simulink model "simQuad"  (R2016a)
settings: Solver=VariableStepAuto  StartTime=0.0  StopTime=10  FixedStep=dt  RelTol=1e-3
values from neighbouring files (symbols this model uses):
  ic = [-3 0 0 0 0 0 0 0 0 0 0 0]    [cf_pid_compare.m]    (also in main.m = [0 0 0 0 0 0 0 0 0 0 0 0])
  Ki = 0.004    [main.m]
  Kp = 0.5    [main.m]
  r2d = 180/pi    (= 57.2957795131)    [main.m]
  T_takeoff = 5    [main.m]
undefined symbols (not defined in the file or in its folder): default_ctl, run_away
undefined symbols (not defined in the file): cf2, geometric_ctl, ic2
libraries: simulink x22, aerolibtransform2 x10, vrlib x8, aerolibutil x5, cstblocks x4, aerolibnav x2, dspmathops x2
(part 1 of 2)
settings Model: Creator=appatte2  LastModifiedBy=arun

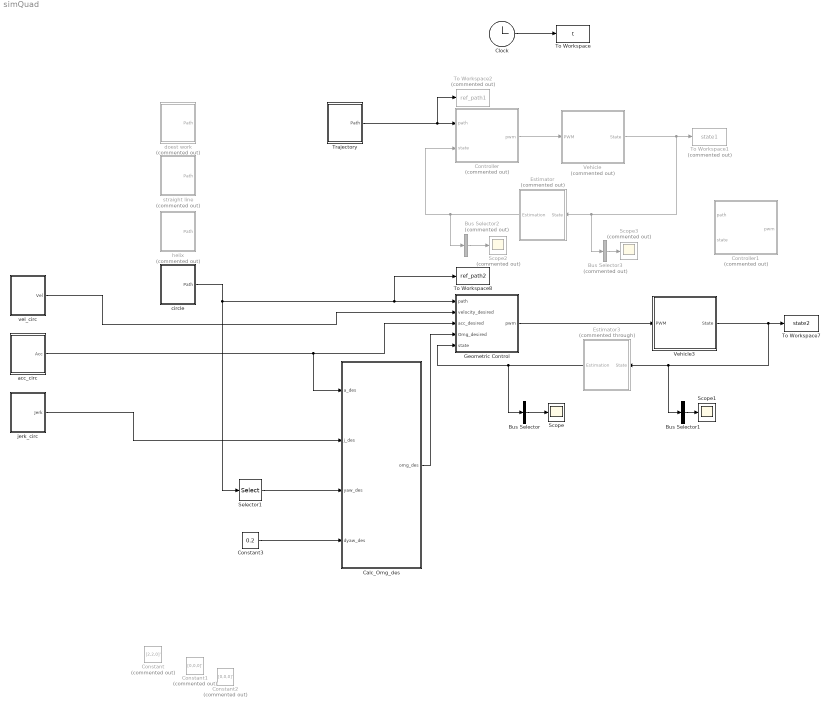
== system simQuad ==
  Bus Selector : BusSelector  OutputSignals=roll,pitch,yaw  OutputAsBus=on
  Bus Selector1 : BusSelector  OutputSignals=roll,pitch,yaw  OutputAsBus=on
  Bus Selector2 : BusSelector  Commented=on  OutputSignals=roll,pitch,yaw  OutputAsBus=on
  Bus Selector3 : BusSelector  Commented=on  OutputSignals=roll,pitch,yaw  OutputAsBus=on
  "Calc_Omg_des " : MATLAB Function  TreatAsAtomicUnit=on
  Clock : Clock
  Constant : Constant  Commented=on  Value=[2,2,0]'
  Constant1 : Constant  Commented=on  Value=[0,0,0]'
  Constant2 : Constant  Commented=on  Value=[0,0,0]'
  Constant3 : Constant  Value=0.2
  Controller : Subsystem  Commented=on  mask(PID Controller for Quadrotor){mix=default_ctl.mix, rates=default_ctl.rates, att=default_ctl.att, pos=default_ctl.pos, sat=default_ctl.sat, intSat=default_ctl.intSat}
      mask prompts: mix "Motor Mixing Table"; rates "Rate Control Table"; att "Attitude Control Table"; pos "Position Control Table"; sat "Attitude Limits"; intSat "Integral Saturation"
      mask help: Allows user to set parameters for pid controllers on rates, angles and linear position.
  Controller1 : Subsystem  Commented=on  mask(PID Controller for Quadrotor){mix=default_ctl.mix, rates=default_ctl.rates, att=default_ctl.att, pos=default_ctl.pos, sat=default_ctl.sat, intSat=default_ctl.intSat}
      mask prompts: mix "Motor Mixing Table"; rates "Rate Control Table"; att "Attitude Control Table"; pos "Position Control Table"; sat "Attitude Limits"; intSat "Integral Saturation"
      mask help: Allows user to set parameters for pid controllers on rates, angles and linear position.
  Estimator : Subsystem  Commented=on  mask{rng_seed=1111}
      mask prompts: rng_seed "Random Seed"
  Estimator3 : Subsystem  Commented=through  mask{rng_seed=1111}
      mask prompts: rng_seed "Random Seed"
  Geometric Control : Subsystem  mask(PID Controller for Quadrotor){model=cf2, ctl=geometric_ctl}
      mask prompts: model "Quad Model"; ctl "Controller"
      mask help: Allows user to set parameters for pid controllers on rates, angles and linear position.
  Scope : Scope
  Scope1 : Scope
  Scope2 : Scope  Commented=on
  Scope3 : Scope  Commented=on
  Selector1 : Selector  InputPortWidth=4  IndexOptions=Index vector (dialog)  Indices=[4]  OutputSizes=1
  To Workspace : ToWorkspace  VariableName=t  SaveFormat=Timeseries  SampleTime=-1
  To Workspace1 : ToWorkspace  Commented=on  VariableName=state1  SampleTime=-1
  To Workspace2 : ToWorkspace  Commented=on  VariableName=ref_path1  SampleTime=-1
      settings: Save2DSignal=2-D array (concatenate along first dimension)
  To Workspace7 : ToWorkspace  VariableName=state2  SampleTime=-1
  To Workspace8 : ToWorkspace  VariableName=ref_path2  SampleTime=-1
      settings: Save2DSignal=2-D array (concatenate along first dimension)
  Trajectory : Subsystem
  Vehicle : Subsystem  Commented=on  mask{model=cf2, ic=ic}
      mask prompts: model "Model Object"; ic "Initial Condition"
  Vehicle3 : Subsystem  mask{model=cf2, ic=ic2}
      mask prompts: model "Model Object"; ic "Initial Condition"
  acc_circ : Subsystem
  "circle " : Subsystem
  doest work : Subsystem  Commented=on
  helix : Subsystem  Commented=on
  jerk_circ : Subsystem
  straight line : Subsystem  Commented=on
  vel_circ : Subsystem
  wires:
  Clock/1 -> To Workspace/1
  Controller/1(pwm) -> Vehicle/1(PWM)
  Geometric Control/1(pwm) -> Vehicle3/1(PWM)
  Trajectory/1(Path) -> To Workspace2/1, Controller/1(path)
  "Calc_Omg_des "/1(omg_des) -> Geometric Control/4(Omg_desired)
  Estimator3/1(Estimation) -> Geometric Control/5(state), Bus Selector/1
  Vehicle3/1(State) -> Estimator3/1(State), Bus Selector1/1, To Workspace7/1
  Bus Selector/1 -> Scope/1
  Bus Selector1/1 -> Scope1/1
  Estimator/1(Estimation) -> Bus Selector2/1, Controller/2(state)
  Bus Selector2/1 -> Scope2/1
  Vehicle/1(State) -> Bus Selector3/1, Estimator/1(State), To Workspace1/1
  Bus Selector3/1 -> Scope3/1
  "circle "/1(Path) -> To Workspace8/1, Geometric Control/1(path), Selector1/1
  Selector1/1 -> "Calc_Omg_des "/3(yaw_des)
  Constant3/1 -> "Calc_Omg_des "/4(dyaw_des)
  vel_circ/1(Vel) -> Geometric Control/2(velocity_desired)
  acc_circ/1(Acc) -> "Calc_Omg_des "/1(a_des), Geometric Control/3("acc_desired ")
  jerk_circ/1(Jerk) -> "Calc_Omg_des "/2(j_des)

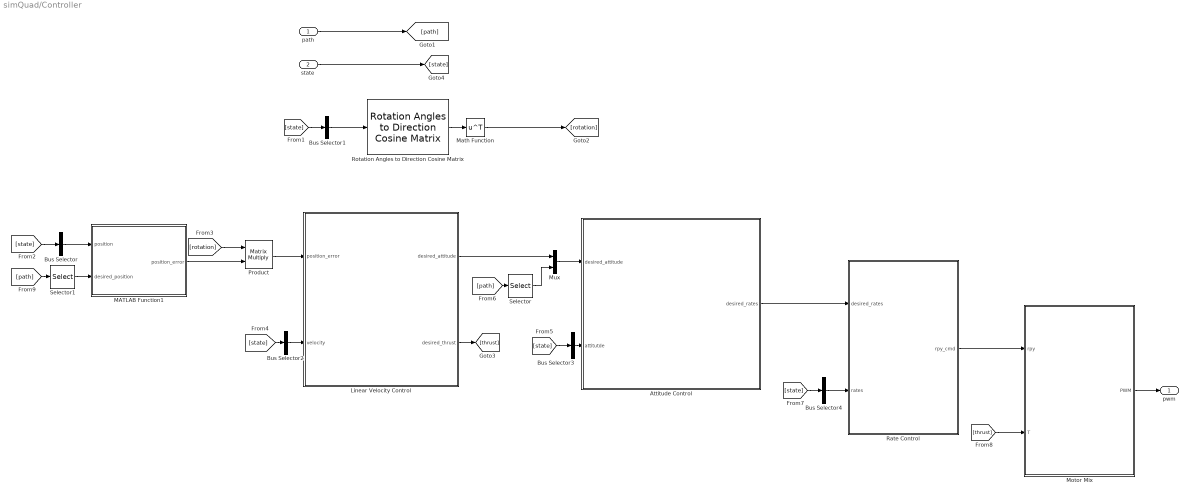
== system simQuad/Controller ==
  path : Inport
  state : Inport  Port=2
  Attitude Control : Subsystem
  Bus Selector : BusSelector  OutputSignals=x,y,z  OutputAsBus=on
  Bus Selector1 : BusSelector  OutputSignals=roll,pitch,yaw  OutputAsBus=on
  Bus Selector2 : BusSelector  OutputSignals=dx,dy,dz  OutputAsBus=on
  Bus Selector3 : BusSelector  OutputSignals=roll,pitch,yaw  OutputAsBus=on
  Bus Selector4 : BusSelector  OutputSignals=droll,dpitch,dyaw  OutputAsBus=on
  Linear Velocity Control : Subsystem
  MATLAB Function1 : MATLAB Function  TreatAsAtomicUnit=on
  Math Function : Math  Operator=transpose  SaturateOnIntegerOverflow=on
  Motor Mix : Subsystem
  Mux : Mux  Inputs=2
  Product : Product  Multiplication=Matrix(*)
  Rate Control : Subsystem
  Rotation Angles to Direction Cosine Matrix : aerolibtransform2/Rotation Angles to Direction Cosine Matrix  rotationOrder=ZYX
  Selector : Selector  InputPortWidth=4  IndexOptions=Index vector (dialog)  Indices=[4]  OutputSizes=1
  Selector1 : Selector  InputPortWidth=4  IndexOptions=Index vector (dialog)  Indices=[1 2 3]  OutputSizes=1
  pwm : Outport
  wires:
  [path] -> Selector1/1
  [state] -> Bus Selector/1
  Motor Mix/1(PWM) -> pwm/1
  Selector1/1 -> MATLAB Function1/2(desired_position)
  Bus Selector/1 -> MATLAB Function1/1(position)
  [rotation] -> Product/1
  Mux/1 -> Attitude Control/1(desired_attitude)
  Bus Selector1/1 -> Rotation Angles to Direction Cosine Matrix/1
  [state] -> Bus Selector3/1
  Bus Selector3/1 -> Attitude Control/2(attitutde)
  Bus Selector2/1 -> Linear Velocity Control/2(velocity)
  [state] -> Bus Selector2/1
  [state] -> Bus Selector1/1
  [thrust] -> Motor Mix/2(T)
  Attitude Control/1(desired_rates) -> Rate Control/1(desired_rates)
  [state] -> Bus Selector4/1
  Bus Selector4/1 -> Rate Control/2(rates)
  [path] -> Selector/1
  Selector/1 -> Mux/2
  Linear Velocity Control/2(desired_thrust) -> [thrust]
  state/1 -> [state]
  path/1 -> [path]
  MATLAB Function1/1(position_error) -> Product/2
  Rotation Angles to Direction Cosine Matrix/1 -> Math Function/1
  Product/1 -> Linear Velocity Control/1(position_error)
  Linear Velocity Control/1(desired_attitude) -> Mux/1
  Math Function/1 -> [rotation]
  Rate Control/1(rpy_cmd) -> Motor Mix/1(rpy)

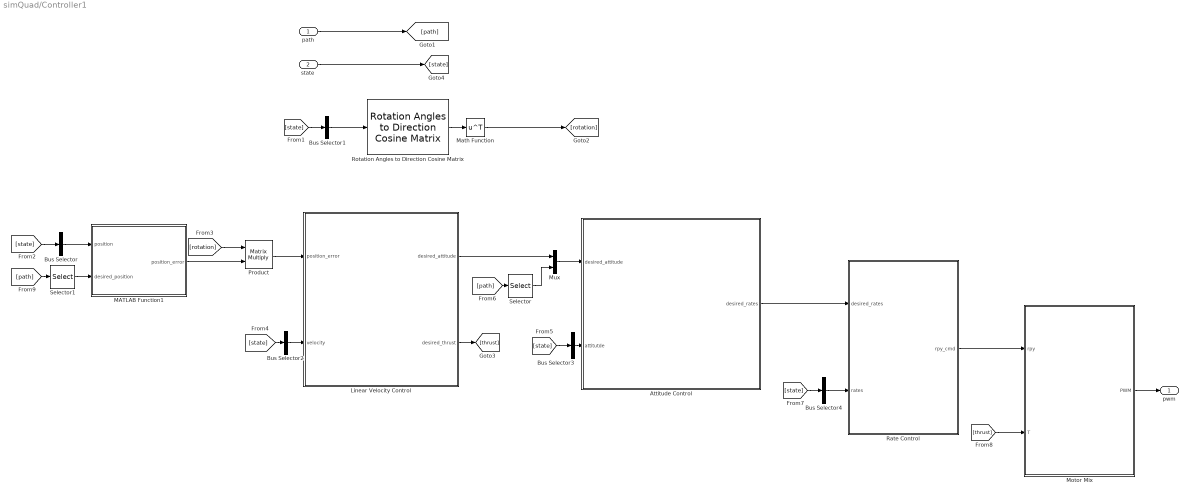
== system simQuad/Controller1 ==
  path : Inport
  state : Inport  Port=2
  Attitude Control : Subsystem
  Bus Selector : BusSelector  OutputSignals=x,y,z  OutputAsBus=on
  Bus Selector1 : BusSelector  OutputSignals=roll,pitch,yaw  OutputAsBus=on
  Bus Selector2 : BusSelector  OutputSignals=dx,dy,dz  OutputAsBus=on
  Bus Selector3 : BusSelector  OutputSignals=roll,pitch,yaw  OutputAsBus=on
  Bus Selector4 : BusSelector  OutputSignals=droll,dpitch,dyaw  OutputAsBus=on
  Linear Velocity Control : Subsystem
  MATLAB Function1 : MATLAB Function  TreatAsAtomicUnit=on
  Math Function : Math  Operator=transpose  SaturateOnIntegerOverflow=on
  Motor Mix : Subsystem
  Mux : Mux  Inputs=2
  Product : Product  Multiplication=Matrix(*)
  Rate Control : Subsystem
  Rotation Angles to Direction Cosine Matrix : aerolibtransform2/Rotation Angles to Direction Cosine Matrix  rotationOrder=ZYX
  Selector : Selector  InputPortWidth=4  IndexOptions=Index vector (dialog)  Indices=[4]  OutputSizes=1
  Selector1 : Selector  InputPortWidth=4  IndexOptions=Index vector (dialog)  Indices=[1 2 3]  OutputSizes=1
  pwm : Outport
  wires:
  [path] -> Selector1/1
  [state] -> Bus Selector/1
  Motor Mix/1(PWM) -> pwm/1
  Selector1/1 -> MATLAB Function1/2(desired_position)
  Bus Selector/1 -> MATLAB Function1/1(position)
  [rotation] -> Product/1
  Mux/1 -> Attitude Control/1(desired_attitude)
  Bus Selector1/1 -> Rotation Angles to Direction Cosine Matrix/1
  [state] -> Bus Selector3/1
  Bus Selector3/1 -> Attitude Control/2(attitutde)
  Bus Selector2/1 -> Linear Velocity Control/2(velocity)
  [state] -> Bus Selector2/1
  [state] -> Bus Selector1/1
  [thrust] -> Motor Mix/2(T)
  Attitude Control/1(desired_rates) -> Rate Control/1(desired_rates)
  [state] -> Bus Selector4/1
  Bus Selector4/1 -> Rate Control/2(rates)
  [path] -> Selector/1
  Selector/1 -> Mux/2
  Linear Velocity Control/2(desired_thrust) -> [thrust]
  state/1 -> [state]
  path/1 -> [path]
  MATLAB Function1/1(position_error) -> Product/2
  Rotation Angles to Direction Cosine Matrix/1 -> Math Function/1
  Product/1 -> Linear Velocity Control/1(position_error)
  Linear Velocity Control/1(desired_attitude) -> Mux/1
  Math Function/1 -> [rotation]
  Rate Control/1(rpy_cmd) -> Motor Mix/1(rpy)

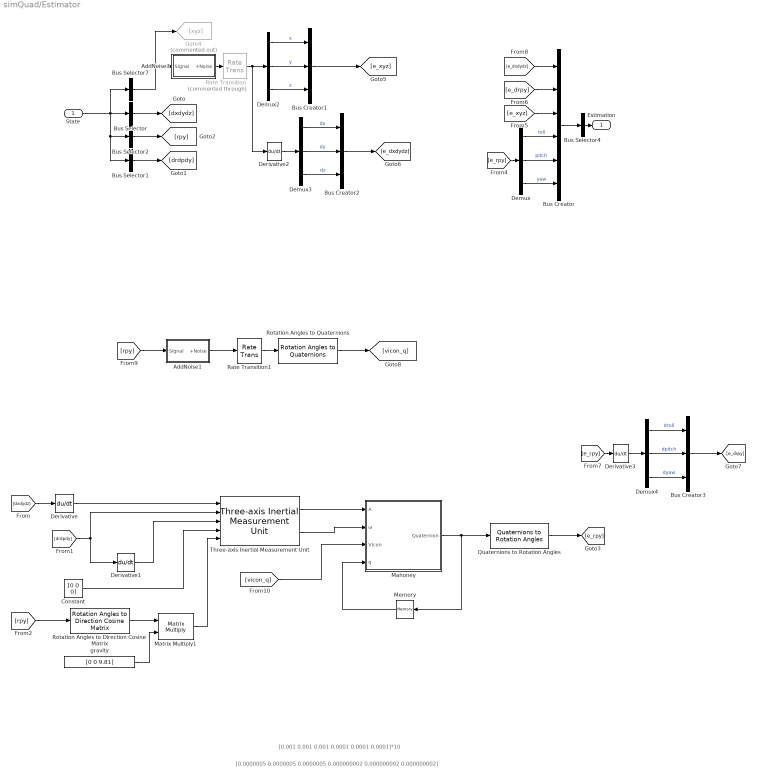
== system simQuad/Estimator ==
  note: [0.001 0.001 0.001 0.0001 0.0001 0.0001]*10
  note: [0.0000005 0.0000005 0.0000005 0.000000002 0.000000002 0.000000002]
  State : Inport
  AddNoise1 : Subsystem
  AddNoise3 : Subsystem
  Bus Creator : BusCreator  Inputs=6
  Bus Creator1 : BusCreator  Inputs=3
  Bus Creator2 : BusCreator  Inputs=3
  Bus Creator3 : BusCreator  Inputs=3
  Bus Selector : BusSelector  OutputSignals=dx,dy,dz  OutputAsBus=on
  Bus Selector1 : BusSelector  OutputSignals=droll,dpitch,dyaw  OutputAsBus=on
  Bus Selector2 : BusSelector  OutputSignals=roll,pitch,yaw  OutputAsBus=on
  Bus Selector4 : BusSelector  OutputSignals=roll,pitch,yaw,signal3.x,signal3.y,signal3.z,signal2.droll,signal2.dpitch,signal2.dyaw,signal1.dx,signal1.dy,signal1.dz  OutputAsBus=on
  Bus Selector7 : BusSelector  OutputSignals=x,y,z  OutputAsBus=on
  Constant : Constant  Value=[0 0 0]
  Demux{,2..4} (4 alike) : Demux  Outputs=3
  Derivative{,1..3} (4 alike) : Derivative
  Goto4 : Goto  Commented=on  GotoTag=xyz
  Mahoney : Subsystem
  Matrix Multiply1 : Product  Multiplication=Matrix(*)
  Memory : Memory  X0=[1 0 0 0]
  Quaternions to Rotation Angles : aerolibtransform2/Quaternions to Rotation Angles  rotationOrder=XYZ
  Rate Transition : RateTransition  Commented=through  OutPortSampleTime=0.005
  Rate Transition1 : RateTransition  OutPortSampleTime=0.005
  Rotation Angles to Direction Cosine Matrix : aerolibtransform2/Rotation Angles to Direction Cosine Matrix  rotationOrder=XYZ
  Rotation Angles to Quaternions : aerolibtransform2/Rotation Angles to Quaternions  rotationOrder=XYZ
  Three-axis Inertial Measurement Unit : aerolibnav/Three-axis Inertial Measurement Unit  units=Metric (MKS)  imu=[0 0 0]  dtype_a=on  w_a=190  z_a=0.707  a_sf_cc=[0.98 0 0; 0 0.98 0; 0 0 0.98]  a_bias=[0 0 0]  a_sat="[-19.62  -19.62  -19.62 19.62 19.62 19.62]"  dtype_g=on  w_g=190  z_g=0.707  g_sf_cc=[.98 0 0; 0 .98 0; 0 0 .98]  g_bias=[0 0 0]  g_sens=[0 0 0]  g_sat="[-4.36  -4.36  -4.36 4.36 4.36 4.36]"  i_rand=on  i_seeds=[23093 23094 23095 23096 23097 23098]*rng_seed  i_pow=[0.001 0.001 0.001 0.0001 0.0001 0.0001]*10  i_Ts=0
  gravity : Constant  Value=[0 0 9.81]
  Estimation : Outport
  wires:
  State/1 -> Bus Selector1/1, Bus Selector2/1, Bus Selector7/1, Bus Selector/1
  Bus Creator/1 -> Bus Selector4/1
  Derivative/1 -> Three-axis Inertial Measurement Unit/1
  Constant/1 -> Three-axis Inertial Measurement Unit/4
  Memory/1 -> Mahoney/4(q)
  Mahoney/1(Quaternion) -> Memory/1, Quaternions to Rotation Angles/1
  Three-axis Inertial Measurement Unit/1 -> Mahoney/1(A)
  Three-axis Inertial Measurement Unit/2 -> Mahoney/2(ω)
  Derivative1/1 -> Three-axis Inertial Measurement Unit/3
  gravity/1 -> Matrix Multiply1/2
  Rotation Angles to Direction Cosine Matrix/1 -> Matrix Multiply1/1
  Matrix Multiply1/1 -> Three-axis Inertial Measurement Unit/5
  Bus Selector/1 -> [dxdydz]
  [dxdydz] -> Derivative/1
  Bus Selector1/1 -> [drdpdy]
  [drdpdy] -> Three-axis Inertial Measurement Unit/2, Derivative1/1
  Bus Selector2/1 -> [rpy]
  [rpy] -> Rotation Angles to Direction Cosine Matrix/1
  Demux/2 -> Bus Creator/5  "pitch"
  Demux/1 -> Bus Creator/4  "roll"
  [e_rpy] -> Demux/1
  Demux/3 -> Bus Creator/6  "yaw"
  Bus Selector4/1 -> Estimation/1
  [e_xyz] -> Bus Creator/3
  [e_drpy] -> Bus Creator/2
  [e_dxdydz] -> Bus Creator/1
  Bus Selector7/1 -> Goto4/1, AddNoise3/1(Signal)
  AddNoise3/1(+Noise) -> Rate Transition/1
  Rate Transition/1 -> Derivative2/1, Demux2/1
  Demux2/1 -> Bus Creator1/1  "x"
  Demux2/3 -> Bus Creator1/3  "z"
  Demux2/2 -> Bus Creator1/2  "y"
  Bus Creator1/1 -> [e_xyz]
  Demux3/3 -> Bus Creator2/3  "dz"
  Derivative2/1 -> Demux3/1
  Demux3/2 -> Bus Creator2/2  "dy"
  Demux3/1 -> Bus Creator2/1  "dx"
  Bus Creator2/1 -> [e_dxdydz]
  Demux4/3 -> Bus Creator3/3  "dyaw"
  Derivative3/1 -> Demux4/1
  Demux4/2 -> Bus Creator3/2  "dpitch"
  Demux4/1 -> Bus Creator3/1  "droll"
  Bus Creator3/1 -> [e_drpy]
  [e_rpy] -> Derivative3/1
  Rotation Angles to Quaternions/1 -> [vicon_q]
  [vicon_q] -> Mahoney/3(Vicon)
  Rate Transition1/1 -> Rotation Angles to Quaternions/1
  AddNoise1/1(+Noise) -> Rate Transition1/1
  [rpy] -> AddNoise1/1(Signal)
  Quaternions to Rotation Angles/1 -> [e_rpy]

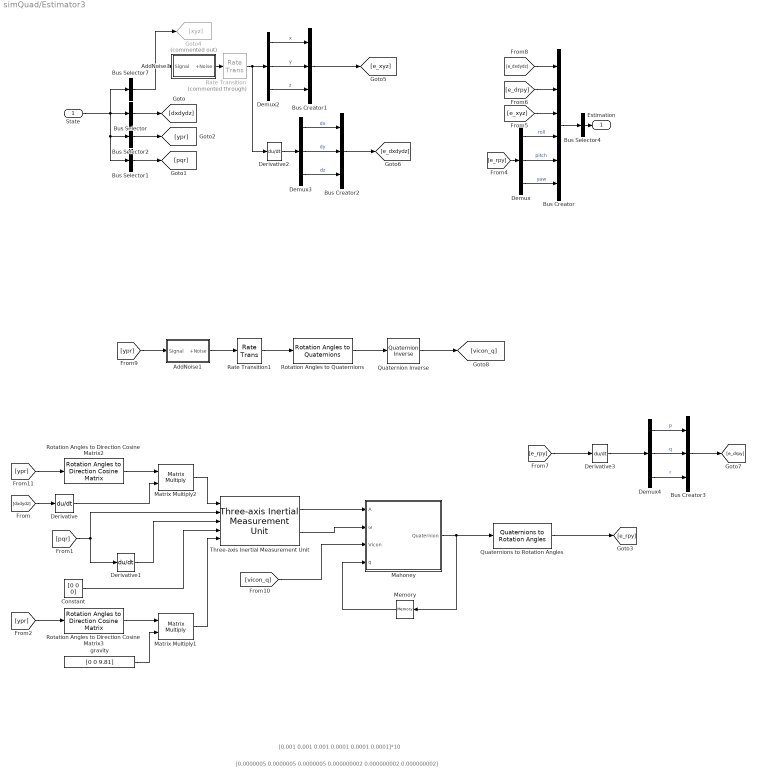
== system simQuad/Estimator3 ==
  note: [0.0000005 0.0000005 0.0000005 0.000000002 0.000000002 0.000000002]
  note: [0.001 0.001 0.001 0.0001 0.0001 0.0001]*10
  State : Inport
  AddNoise1 : Subsystem
  AddNoise3 : Subsystem
  Bus Creator : BusCreator  Inputs=6
  Bus Creator1 : BusCreator  Inputs=3
  Bus Creator2 : BusCreator  Inputs=3
  Bus Creator3 : BusCreator  Inputs=3
  Bus Selector : BusSelector  OutputSignals=dx,dy,dz  OutputAsBus=on
  Bus Selector1 : BusSelector  OutputSignals=p,q,r  OutputAsBus=on
  Bus Selector2 : BusSelector  OutputSignals=yaw,pitch,roll  OutputAsBus=on
  Bus Selector4 : BusSelector  OutputSignals=roll,pitch,yaw,signal3.x,signal3.y,signal3.z,signal2.p,signal2.q,signal2.r,signal1.dx,signal1.dy,signal1.dz  OutputAsBus=on
  Bus Selector7 : BusSelector  OutputSignals=x,y,z  OutputAsBus=on
  Constant : Constant  Value=[0 0 0]
  Demux{,2..4} (4 alike) : Demux  Outputs=3
  Derivative{,1..3} (4 alike) : Derivative
  Goto4 : Goto  Commented=on  GotoTag=xyz
  Mahoney : Subsystem
  Matrix Multiply1 : Product  Multiplication=Matrix(*)
  Matrix Multiply2 : Product  Multiplication=Matrix(*)
  Memory : Memory  X0=[1 0 0 0]
  Quaternion Inverse : aerolibutil/Quaternion Inverse
  Quaternions to Rotation Angles : aerolibtransform2/Quaternions to Rotation Angles  rotationOrder=XYZ
  Rate Transition : RateTransition  Commented=through  OutPortSampleTime=0.005
  Rate Transition1 : RateTransition  OutPortSampleTime=0.005
  Rotation Angles to Direction Cosine Matrix2 : aerolibtransform2/Rotation Angles to Direction Cosine Matrix  rotationOrder=ZYX
  Rotation Angles to Direction Cosine Matrix3 : aerolibtransform2/Rotation Angles to Direction Cosine Matrix  rotationOrder=ZYX
  Rotation Angles to Quaternions : aerolibtransform2/Rotation Angles to Quaternions  rotationOrder=ZYX
  Three-axis Inertial Measurement Unit : aerolibnav/Three-axis Inertial Measurement Unit  units=Metric (MKS)  imu=[0 0 0]  dtype_a=on  w_a=190  z_a=0.707  a_sf_cc=[0.98 0 0; 0 0.98 0; 0 0 0.98]  a_bias=[0 0 0]  a_sat="[-19.62  -19.62  -19.62 19.62 19.62 19.62]"  dtype_g=on  w_g=190  z_g=0.707  g_sf_cc=[.98 0 0; 0 .98 0; 0 0 .98]  g_bias=[0 0 0]  g_sens=[0 0 0]  g_sat="[-4.36  -4.36  -4.36 4.36 4.36 4.36]"  i_rand=on  i_seeds=[23093 23094 23095 23096 23097 23098]*rng_seed  i_pow=[0.001 0.001 0.001 0.0001 0.0001 0.0001]*10  i_Ts=0
  gravity : Constant  Value=[0 0 9.81]
  Estimation : Outport
  wires:
  [ypr] -> AddNoise1/1(Signal)
  AddNoise1/1(+Noise) -> Rate Transition1/1
  Rate Transition1/1 -> Rotation Angles to Quaternions/1
  [vicon_q] -> Mahoney/3(Vicon)
  [e_rpy] -> Derivative3/1
  Bus Creator3/1 -> [e_drpy]
  Demux4/1 -> Bus Creator3/1  "p"
  Demux4/2 -> Bus Creator3/2  "q"
  Derivative3/1 -> Demux4/1
  Demux4/3 -> Bus Creator3/3  "r"
  Bus Creator2/1 -> [e_dxdydz]
  Demux3/1 -> Bus Creator2/1  "dx"
  Demux3/2 -> Bus Creator2/2  "dy"
  Derivative2/1 -> Demux3/1
  Demux3/3 -> Bus Creator2/3  "dz"
  Bus Creator1/1 -> [e_xyz]
  Demux2/2 -> Bus Creator1/2  "y"
  Demux2/3 -> Bus Creator1/3  "z"
  Demux2/1 -> Bus Creator1/1  "x"
  Rate Transition/1 -> Demux2/1, Derivative2/1
  AddNoise3/1(+Noise) -> Rate Transition/1
  Bus Selector7/1 -> AddNoise3/1(Signal), Goto4/1
  [e_dxdydz] -> Bus Creator/1
  [e_drpy] -> Bus Creator/2
  [e_xyz] -> Bus Creator/3
  Bus Selector4/1 -> Estimation/1
  Demux/3 -> Bus Creator/6  "yaw"
  [e_rpy] -> Demux/1
  Demux/1 -> Bus Creator/4  "roll"
  Demux/2 -> Bus Creator/5  "pitch"
  Bus Selector2/1 -> [ypr]
  [pqr] -> Derivative1/1, Three-axis Inertial Measurement Unit/2
  Bus Selector1/1 -> [pqr]
  [dxdydz] -> Derivative/1
  Bus Selector/1 -> [dxdydz]
  Matrix Multiply1/1 -> Three-axis Inertial Measurement Unit/5
  Rotation Angles to Direction Cosine Matrix3/1 -> Matrix Multiply1/1
  gravity/1 -> Matrix Multiply1/2
  Derivative1/1 -> Three-axis Inertial Measurement Unit/3
  Three-axis Inertial Measurement Unit/2 -> Mahoney/2(ω)
  Three-axis Inertial Measurement Unit/1 -> Mahoney/1(A)
  Memory/1 -> Mahoney/4(q)
  Constant/1 -> Three-axis Inertial Measurement Unit/4
  Derivative/1 -> Matrix Multiply2/2
  Bus Creator/1 -> Bus Selector4/1
  State/1 -> Bus Selector/1, Bus Selector7/1, Bus Selector2/1, Bus Selector1/1
  Matrix Multiply2/1 -> Three-axis Inertial Measurement Unit/1
  Rotation Angles to Direction Cosine Matrix2/1 -> Matrix Multiply2/1
  [ypr] -> Rotation Angles to Direction Cosine Matrix2/1
  [ypr] -> Rotation Angles to Direction Cosine Matrix3/1
  Rotation Angles to Quaternions/1 -> Quaternion Inverse/1
  Mahoney/1(Quaternion) -> Quaternions to Rotation Angles/1, Memory/1
  Quaternions to Rotation Angles/1 -> [e_rpy]
  Quaternion Inverse/1 -> [vicon_q]

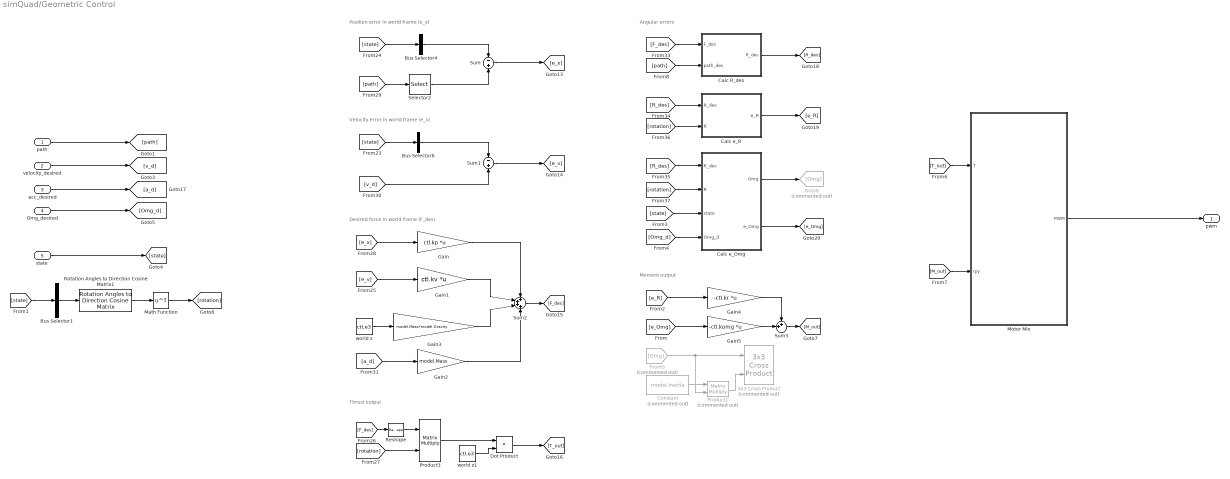
== system simQuad/Geometric Control ==
  note: Moment output
  note: Angular errors
  note: Thrust output
  note: Desired force in world frame (F_des)
  note: Velocity error in world frame (e_v)
  note: Position error in world frame (e_x)
  path : Inport
  velocity_desired : Inport  Port=2
  "acc_desired " : Inport  Port=3
  Omg_desired : Inport  Port=4
  state : Inport  Port=5
  3x3 Cross Product : aerolibutil/3x3 Cross Product  Commented=on
  Bus Selector1 : BusSelector  OutputSignals=yaw,pitch,roll  OutputAsBus=on
  Bus Selector4 : BusSelector  OutputSignals=x,y,z  OutputAsBus=on
  Bus Selector6 : BusSelector  OutputSignals=dx,dy,dz  OutputAsBus=on
  Calc R_des : Subsystem
  Calc e_Omg : Subsystem
  Calc e_R : Subsystem
  Constant : Constant  Commented=on  Value=model.Inertia
  Dot Product : DotProduct  InputSameDT=on  OutDataTypeStr=Inherit: Inherit via internal rule
  From5 : From  Commented=on  GotoTag=Omg
  Gain : Gain  Gain=ctl.kp  Multiplication=Matrix(K*u) (u vector)
  Gain1 : Gain  Gain=ctl.kv  Multiplication=Matrix(K*u) (u vector)
  Gain2 : Gain  Gain=model.Mass
  Gain3 : Gain  Gain=model.Mass*model.Gravity
  Gain4 : Gain  Gain=-ctl.kr  Multiplication=Matrix(K*u) (u vector)
  Gain5 : Gain  Gain=-ctl.komg  Multiplication=Matrix(K*u) (u vector)
  Goto6 : Goto  Commented=on  GotoTag=Omg
  Math Function : Math  Operator=transpose  SaturateOnIntegerOverflow=on
  Motor Mix : Subsystem
  Product1 : Product  Commented=on  Multiplication=Matrix(*)
  Product3 : Product  Multiplication=Matrix(*)
  Reshape : Reshape  OutputDimensionality=Row vector (2-D)
  Rotation Angles to Direction Cosine Matrix1 : aerolibtransform2/Rotation Angles to Direction Cosine Matrix  rotationOrder=ZYX
  Selector2 : Selector  InputPortWidth=4  IndexOptions=Index vector (dialog)  Indices=[1 2 3]  OutputSizes=1
  Sum : Sum  Inputs=-|+
  Sum1 : Sum  Inputs=-|+
  Sum2 : Sum  Inputs=++++
  Sum3 : Sum  Inputs=++|
  world z : Constant  Value=ctl.e3
  world z1 : Constant  Value=ctl.e3
  pwm : Outport
  wires:
  state/1 -> [state]
  path/1 -> [path]
  velocity_desired/1 -> [v_d]
  Motor Mix/1(PWM) -> pwm/1
  [path] -> Selector2/1
  [state] -> Bus Selector4/1
  Bus Selector4/1 -> Sum/1
  [state] -> Bus Selector6/1
  Sum1/1 -> [e_v]
  [v_d] -> Sum1/2
  [e_x] -> Gain/1
  [e_v] -> Gain1/1
  [a_d] -> Gain2/1
  world z/1 -> Gain3/1
  Gain3/1 -> Sum2/3
  Gain2/1 -> Sum2/4
  Gain1/1 -> Sum2/2
  Gain/1 -> Sum2/1
  Sum2/1 -> [F_des]
  [F_des] -> Reshape/1
  Product3/1 -> Dot Product/1
  "acc_desired "/1 -> [a_d]
  [F_des] -> Calc R_des/1(F_des)
  [path] -> Calc R_des/2(path_des)
  Calc R_des/1(R_des) -> [R_des]
  [R_des] -> Calc e_R/1(R_des)
  [rotation] -> Calc e_R/2(R)
  Calc e_R/1(e_R) -> [e_R]
  [R_des] -> Calc e_Omg/1(R_des)
  [rotation] -> Calc e_Omg/2(R)
  Calc e_Omg/2(e_Omg) -> [e_Omg]
  Omg_desired/1 -> [Omg_d]
  [state] -> Calc e_Omg/3(state)
  [Omg_d] -> Calc e_Omg/4(Omg_d)
  Calc e_Omg/1(Omg) -> Goto6/1
  From5/1 -> 3x3 Cross Product/1, Product1/2
  Constant/1 -> Product1/1
  Product1/1 -> 3x3 Cross Product/2
  [e_R] -> Gain4/1
  [e_Omg] -> Gain5/1
  Gain4/1 -> Sum3/1
  Gain5/1 -> Sum3/2
  [T_out] -> Motor Mix/1(T)
  [M_out] -> Motor Mix/2(rpy)
  Sum/1 -> [e_x]
  Selector2/1 -> Sum/2
  Dot Product/1 -> [T_out]
  [rotation] -> Product3/2
  world z1/1 -> Dot Product/2
  Reshape/1 -> Product3/1
  Bus Selector6/1 -> Sum1/1
  Sum3/1 -> [M_out]
  Rotation Angles to Direction Cosine Matrix1/1 -> Math Function/1
  [state] -> Bus Selector1/1
  Math Function/1 -> [rotation]
  Bus Selector1/1 -> Rotation Angles to Direction Cosine Matrix1/1

== system simQuad/Trajectory ==
  note: X
      | Y
      | Z
      | Yaw
  Constant : Constant  Value=10
  Constant5 : Constant  Value=pi/4
  Gain : Gain  Commented=through  Gain=0
  Gain1 : Gain  Commented=through  Gain=0
  Mux : Mux
  Ramp : simulink/Sources/Ramp  slope=2  start=0  X0=0
  Ramp1 : simulink/Sources/Ramp  slope=2  start=0  X0=0
  Path : Outport
  wires:
  Mux/1 -> Path/1
  Constant5/1 -> Mux/4
  Constant/1 -> Mux/3
  Ramp/1 -> Gain1/1
  Ramp1/1 -> Gain/1
  Gain/1 -> Mux/2
  Gain1/1 -> Mux/1

== system simQuad/Vehicle ==
  PWM : Inport
  PWM 2 Speed : Subsystem
  Vehicle Dynamics : Subsystem
  State : Outport
  wires:
  Vehicle Dynamics/1(State) -> State/1
  PWM/1 -> PWM 2 Speed/1(PWM)
  PWM 2 Speed/1(Omega) -> Vehicle Dynamics/1(Omega)

== system simQuad/Vehicle3 ==
  PWM : Inport
  PWM 2 Speed : Subsystem
  Vehicle Dynamics : Subsystem
  State : Outport
  wires:
  PWM 2 Speed/1(Omega) -> Vehicle Dynamics/1(Omega)
  PWM/1 -> PWM 2 Speed/1(PWM)
  Vehicle Dynamics/1(State) -> State/1

== system simQuad/acc_circ ==
  note: X
      | Y
      | Z
  Constant : Constant  Value=0
  Mux : Mux  Inputs=3
  Sine Wave1 : Sin  Amplitude=3*0.2*0.2  Frequency=.2  Phase=3*pi/2  SampleTime=0
  Sine Wave2 : Sin  Amplitude=3*0.2*0.2  Frequency=.2  Phase=pi  SampleTime=0
  Acc : Outport
  wires:
  Constant/1 -> Mux/3
  Sine Wave2/1 -> Mux/1
  Sine Wave1/1 -> Mux/2
  Mux/1 -> Acc/1

== system simQuad/circle  ==
  note: X
      | Y
      | Z
      | Yaw
  Constant : Constant  Value=10
  Mux : Mux
  Ramp : simulink/Sources/Ramp  slope=0.2  start=0  X0=0
  Sine Wave1 : Sin  Amplitude=3  Frequency=.2  Phase=pi/2  SampleTime=0
  Sine Wave2 : Sin  Amplitude=3  Frequency=.2  SampleTime=0
  Path : Outport
  wires:
  Constant/1 -> Mux/3
  Sine Wave2/1 -> Mux/1
  Sine Wave1/1 -> Mux/2
  Mux/1 -> Path/1
  Ramp/1 -> Mux/4

== system simQuad/doest work ==
  note: X
      | Y
      | Z
      | Yaw
  Add1 : Sum
  Add2 : Sum
  Add3 : Sum
  Constant : Constant  Commented=on  Value=0
  Constant1 : Constant  Commented=on  Value=0
  Constant4 : Constant  Value=10
  Constant5 : Constant  Value=0
  DelayStart : Subsystem  Commented=on
  Mux : Mux
  Ramp : simulink/Sources/Ramp  slope=run_away  start=0  X0=0
  Ramp1 : simulink/Sources/Ramp  slope=-run_away  start=0  X0=0
  Sine Wave1 : Sin  Amplitude=5  Frequency=.5  Phase=pi/2  SampleTime=0
  Sine Wave2 : Sin  Amplitude=5  Frequency=.5  Phase=pi/2  SampleTime=0
  Sine Wave3 : Sin  Amplitude=2  Frequency=.5  Phase=pi/2  SampleTime=0
  Subsystem : Subsystem  Commented=on
  Path : Outport
  wires:
  Add1/1 -> Mux/2
  Add2/1 -> Mux/1
  Constant5/1 -> Mux/4
  Mux/1 -> Path/1
  Constant1/1 -> DelayStart/1(In1)
  DelayStart/1(Out1) -> Subsystem/Enable
  Ramp1/1 -> Add1/1
  Sine Wave1/1 -> Add1/2
  Ramp/1 -> Add2/1
  Sine Wave2/1 -> Add2/2
  Add3/1 -> Mux/3
  Constant4/1 -> Add3/1
  Sine Wave3/1 -> Add3/2

== system simQuad/helix ==
  note: X
      | Y
      | Z
      | Yaw
  Constant5 : Constant  Value=0
  Mux : Mux
  Ramp : simulink/Sources/Ramp  slope=.25  start=0  X0=0
  Sine Wave1 : Sin  Amplitude=3  Frequency=.2  Phase=pi/2  SampleTime=0
  Sine Wave2 : Sin  Amplitude=3  Frequency=.2  SampleTime=0
  Path : Outport
  wires:
  Sine Wave1/1 -> Mux/3
  Sine Wave2/1 -> Mux/1
  Ramp/1 -> Mux/2
  Constant5/1 -> Mux/4
  Mux/1 -> Path/1

== system simQuad/jerk_circ ==
  note: X
      | Y
      | Z
  Constant : Constant  Value=0
  Mux : Mux  Inputs=3
  Sine Wave1 : Sin  Amplitude=3*0.2*0.2  Frequency=.2  SampleTime=0
  Sine Wave2 : Sin  Amplitude=3*0.2*0.2*0.2  Frequency=.2  Phase=3*pi/2  SampleTime=0
  Jerk : Outport
  wires:
  Constant/1 -> Mux/3
  Sine Wave2/1 -> Mux/1
  Sine Wave1/1 -> Mux/2
  Mux/1 -> Jerk/1

== system simQuad/straight line ==
  note: X
      | Y
      | Z
      | Yaw
  Constant : Constant  Commented=on  Value=0
  Constant1 : Constant  Commented=on  Value=0
  Constant2 : Constant
  Constant3 : Constant
  Constant4 : Constant  Value=10
  Constant5 : Constant  Value=0
  DelayStart : Subsystem  Commented=on
  Mux : Mux
  Subsystem : Subsystem  Commented=on
  Subsystem1 : Subsystem
  Subsystem2 : Subsystem
  Path : Outport
  wires:
  Subsystem2/1(Out1) -> Mux/2
  Subsystem1/1(Out1) -> Mux/1
  Constant4/1 -> Mux/3
  Constant5/1 -> Mux/4
  Constant3/1 -> Subsystem1/1(In1)
  Constant2/1 -> Subsystem2/1(In1)
  Mux/1 -> Path/1
  Constant1/1 -> DelayStart/1(In1)
  DelayStart/1(Out1) -> Subsystem/Enable

== system simQuad/vel_circ ==
  note: X
      | Y
      | Z
  Constant : Constant  Value=0
  Mux : Mux  Inputs=3
  Sine Wave1 : Sin  Amplitude=3*0.2  Frequency=.2  Phase=pi  SampleTime=0
  Sine Wave2 : Sin  Amplitude=3*0.2  Frequency=.2  Phase=pi/2  SampleTime=0
  Vel : Outport
  wires:
  Constant/1 -> Mux/3
  Sine Wave2/1 -> Mux/1
  Sine Wave1/1 -> Mux/2
  Mux/1 -> Vel/1

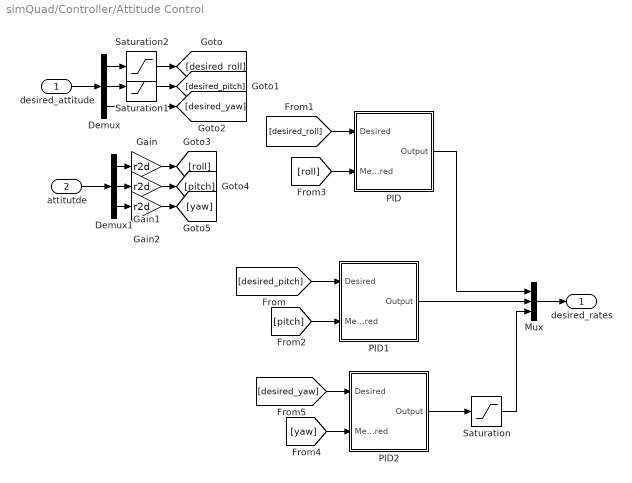
== system simQuad/Controller/Attitude Control ==
  desired_attitude : Inport
  attitutde : Inport  Port=2
  Demux : Demux  Outputs=3
  Demux1 : Demux  Outputs=3
  Gain : Gain  Gain=r2d
  Gain1 : Gain  Gain=r2d
  Gain2 : Gain  Gain=r2d
  Mux : Mux  Inputs=3
  PID : Subsystem
  PID1 : Subsystem
  PID2 : Subsystem
  Saturation : Saturate  UpperLimit=sat(3)  LowerLimit=-sat(3)
  Saturation1 : Saturate  UpperLimit=sat(2)  LowerLimit=-sat(2)
  Saturation2 : Saturate  UpperLimit=sat(1)  LowerLimit=-sat(1)
  desired_rates : Outport
  wires:
  [pitch] -> PID1/2(Measured)
  [desired_pitch] -> PID1/1(Desired)
  [desired_roll] -> PID/1(Desired)
  [roll] -> PID/2(Measured)
  desired_attitude/1 -> Demux/1
  Demux/1 -> Saturation2/1
  Demux/2 -> Saturation1/1
  Demux/3 -> [desired_yaw]
  attitutde/1 -> Demux1/1
  Demux1/1 -> Gain/1
  Demux1/2 -> Gain1/1
  Demux1/3 -> Gain2/1
  [yaw] -> PID2/2(Measured)
  Gain/1 -> [roll]
  Gain1/1 -> [pitch]
  Gain2/1 -> [yaw]
  [desired_yaw] -> PID2/1(Desired)
  PID/1(Output) -> Mux/1
  PID2/1(Output) -> Saturation/1
  PID1/1(Output) -> Mux/2
  Mux/1 -> desired_rates/1
  Saturation/1 -> Mux/3
  Saturation1/1 -> [desired_pitch]
  Saturation2/1 -> [desired_roll]

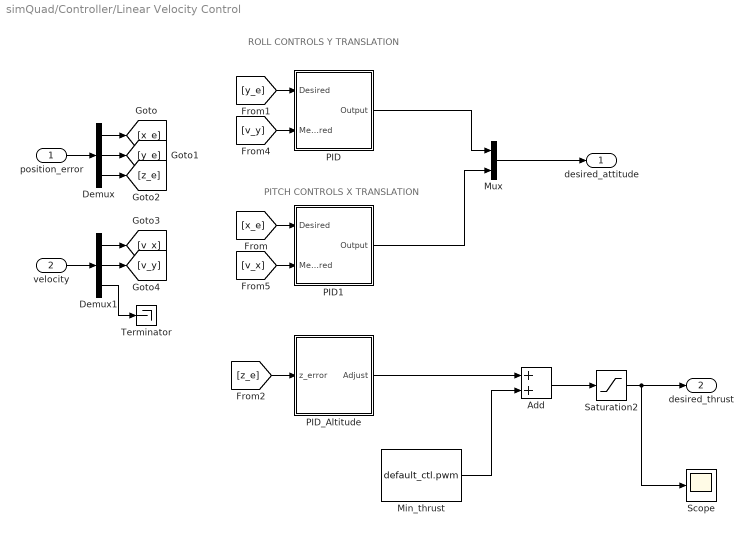
== system simQuad/Controller/Linear Velocity Control ==
  note: ROLL CONTROLS Y TRANSLATION
  note: PITCH CONTROLS X TRANSLATION
  position_error : Inport
  velocity : Inport  Port=2
  Add : Sum
  Demux : Demux  Outputs=3
  Demux1 : Demux  Outputs=3
  "Min_thrust " : Constant  Value=default_ctl.pwm  SampleTime=0
  Mux : Mux  Inputs=2
  PID : Subsystem
  PID1 : Subsystem
  PID_Altitude : Subsystem
  Saturation2 : Saturate  UpperLimit=default_ctl.sat(4,1)  LowerLimit=0
  Scope : Scope
  Terminator : Terminator
  desired_attitude : Outport
  desired_thrust : Outport  Port=2
  wires:
  [y_e] -> PID/1(Desired)
  Saturation2/1 -> Scope/1, desired_thrust/1
  "Min_thrust "/1 -> Add/2
  Add/1 -> Saturation2/1
  PID_Altitude/1(Adjust) -> Add/1
  position_error/1 -> Demux/1
  Demux/1 -> [x_e]
  Demux/2 -> [y_e]
  Demux/3 -> [z_e]
  [z_e] -> PID_Altitude/1(z_error)
  velocity/1 -> Demux1/1
  Demux1/1 -> [v_x]
  Demux1/2 -> [v_y]
  Demux1/3 -> Terminator/1
  [v_y] -> PID/2(Measured)
  Mux/1 -> desired_attitude/1
  PID/1(Output) -> Mux/1
  [x_e] -> PID1/1(Desired)
  [v_x] -> PID1/2(Measured)
  PID1/1(Output) -> Mux/2

== system simQuad/Controller/Motor Mix ==
  rpy : Inport
  T : Inport  Port=2
  Constant : Constant  Value=mix
  Demux : Demux  Outputs=3
  Mux : Mux
  Product : Product  Multiplication=Matrix(*)
  PWM : Outport
  wires:
  T/1 -> Mux/4
  Mux/1 -> Product/2
  Product/1 -> PWM/1
  Constant/1 -> Product/1
  rpy/1 -> Demux/1
  Demux/2 -> Mux/2
  Demux/1 -> Mux/1
  Demux/3 -> Mux/3

== system simQuad/Controller/Rate Control ==
  note: roll
      | pitch
      | yaw
  desired_rates : Inport
  rates : Inport  Port=2
  Demux : Demux  Outputs=3
  Demux1 : Demux  Outputs=3
  Gain : Gain  Gain=r2d
  Gain1 : Gain  Gain=r2d
  Gain2 : Gain  Gain=r2d
  Mux : Mux  Inputs=3
  PID : Subsystem
  PID1 : Subsystem
  PID2 : Subsystem
  rpy_cmd : Outport
  wires:
  desired_rates/1 -> Demux/1
  Demux/1 -> [desired_droll]
  Demux/2 -> [desired_dpitch]
  Demux/3 -> [desired_dyaw]
  rates/1 -> Demux1/1
  Demux1/1 -> Gain/1
  Demux1/2 -> Gain1/1
  Demux1/3 -> Gain2/1
  Gain/1 -> [droll]
  Gain1/1 -> [dpitch]
  Gain2/1 -> [dyaw]
  PID2/1(Output) -> Mux/3
  PID1/1(Output) -> Mux/2
  PID/1(Output) -> Mux/1
  Mux/1 -> rpy_cmd/1
  [desired_dyaw] -> PID2/1(Desired)
  [desired_droll] -> PID/1(Desired)
  [desired_dpitch] -> PID1/1(Desired)
  [dpitch] -> PID1/2(Measured)
  [droll] -> PID/2(Measured)
  [dyaw] -> PID2/2(Measured)

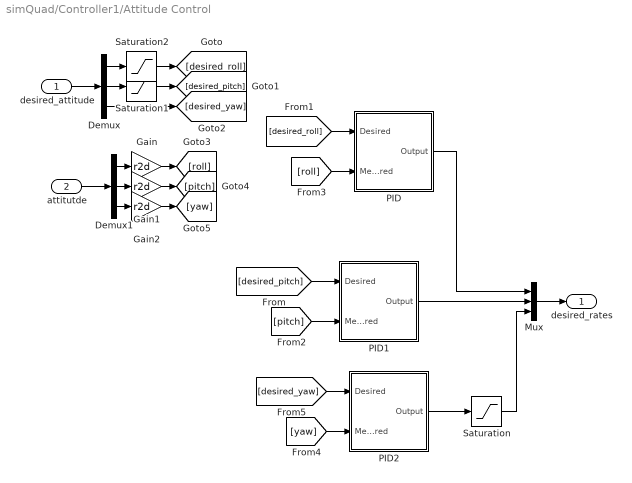
== system simQuad/Controller1/Attitude Control ==
  desired_attitude : Inport
  attitutde : Inport  Port=2
  Demux : Demux  Outputs=3
  Demux1 : Demux  Outputs=3
  Gain : Gain  Gain=r2d
  Gain1 : Gain  Gain=r2d
  Gain2 : Gain  Gain=r2d
  Mux : Mux  Inputs=3
  PID : Subsystem
  PID1 : Subsystem
  PID2 : Subsystem
  Saturation : Saturate  UpperLimit=sat(3)  LowerLimit=-sat(3)
  Saturation1 : Saturate  UpperLimit=sat(2)  LowerLimit=-sat(2)
  Saturation2 : Saturate  UpperLimit=sat(1)  LowerLimit=-sat(1)
  desired_rates : Outport
  wires:
  [pitch] -> PID1/2(Measured)
  [desired_pitch] -> PID1/1(Desired)
  [desired_roll] -> PID/1(Desired)
  [roll] -> PID/2(Measured)
  desired_attitude/1 -> Demux/1
  Demux/1 -> Saturation2/1
  Demux/2 -> Saturation1/1
  Demux/3 -> [desired_yaw]
  attitutde/1 -> Demux1/1
  Demux1/1 -> Gain/1
  Demux1/2 -> Gain1/1
  Demux1/3 -> Gain2/1
  [yaw] -> PID2/2(Measured)
  Gain/1 -> [roll]
  Gain1/1 -> [pitch]
  Gain2/1 -> [yaw]
  [desired_yaw] -> PID2/1(Desired)
  PID/1(Output) -> Mux/1
  PID2/1(Output) -> Saturation/1
  PID1/1(Output) -> Mux/2
  Mux/1 -> desired_rates/1
  Saturation/1 -> Mux/3
  Saturation1/1 -> [desired_pitch]
  Saturation2/1 -> [desired_roll]

== system simQuad/Controller1/Linear Velocity Control ==
  note: ROLL CONTROLS Y TRANSLATION
  note: PITCH CONTROLS X TRANSLATION
  position_error : Inport
  velocity : Inport  Port=2
  Add : Sum
  Demux : Demux  Outputs=3
  Demux1 : Demux  Outputs=3
  "Min_thrust " : Constant  Value=default_ctl.pwm  SampleTime=0
  Mux : Mux  Inputs=2
  PID : Subsystem
  PID1 : Subsystem
  PID_Altitude : Subsystem
  Saturation2 : Saturate  UpperLimit=default_ctl.sat(4,1)  LowerLimit=0
  Terminator : Terminator
  desired_attitude : Outport
  desired_thrust : Outport  Port=2
  wires:
  [y_e] -> PID/1(Desired)
  Saturation2/1 -> desired_thrust/1
  "Min_thrust "/1 -> Add/2
  Add/1 -> Saturation2/1
  PID_Altitude/1(Adjust) -> Add/1
  position_error/1 -> Demux/1
  Demux/1 -> [x_e]
  Demux/2 -> [y_e]
  Demux/3 -> [z_e]
  [z_e] -> PID_Altitude/1(z_error)
  velocity/1 -> Demux1/1
  Demux1/1 -> [v_x]
  Demux1/2 -> [v_y]
  Demux1/3 -> Terminator/1
  [v_y] -> PID/2(Measured)
  Mux/1 -> desired_attitude/1
  PID/1(Output) -> Mux/1
  [x_e] -> PID1/1(Desired)
  [v_x] -> PID1/2(Measured)
  PID1/1(Output) -> Mux/2

== system simQuad/Controller1/Motor Mix ==
  rpy : Inport
  T : Inport  Port=2
  Constant : Constant  Value=mix
  Demux : Demux  Outputs=3
  Mux : Mux
  Product : Product  Multiplication=Matrix(*)
  PWM : Outport
  wires:
  T/1 -> Mux/4
  Mux/1 -> Product/2
  Product/1 -> PWM/1
  Constant/1 -> Product/1
  rpy/1 -> Demux/1
  Demux/2 -> Mux/2
  Demux/1 -> Mux/1
  Demux/3 -> Mux/3

== system simQuad/Controller1/Rate Control ==
  note: roll
      | pitch
      | yaw
  desired_rates : Inport
  rates : Inport  Port=2
  Demux : Demux  Outputs=3
  Demux1 : Demux  Outputs=3
  Gain : Gain  Gain=r2d
  Gain1 : Gain  Gain=r2d
  Gain2 : Gain  Gain=r2d
  Mux : Mux  Inputs=3
  PID : Subsystem
  PID1 : Subsystem
  PID2 : Subsystem
  rpy_cmd : Outport
  wires:
  desired_rates/1 -> Demux/1
  Demux/1 -> [desired_droll]
  Demux/2 -> [desired_dpitch]
  Demux/3 -> [desired_dyaw]
  rates/1 -> Demux1/1
  Demux1/1 -> Gain/1
  Demux1/2 -> Gain1/1
  Demux1/3 -> Gain2/1
  Gain/1 -> [droll]
  Gain1/1 -> [dpitch]
  Gain2/1 -> [dyaw]
  PID2/1(Output) -> Mux/3
  PID1/1(Output) -> Mux/2
  PID/1(Output) -> Mux/1
  Mux/1 -> rpy_cmd/1
  [desired_dyaw] -> PID2/1(Desired)
  [desired_droll] -> PID/1(Desired)
  [desired_dpitch] -> PID1/1(Desired)
  [dpitch] -> PID1/2(Measured)
  [droll] -> PID/2(Measured)
  [dyaw] -> PID2/2(Measured)

== system simQuad/Estimator/AddNoise1 ==
  Signal : Inport
  AddNoise : Subsystem
  AddNoise1 : Subsystem
  AddNoise2 : Subsystem
  Demux : Demux  Outputs=3
  Mux : Mux  Inputs=3
  +Noise : Outport
  wires:
  Mux/1 -> +Noise/1
  Signal/1 -> Demux/1
  AddNoise2/1(+Noise) -> Mux/3
  AddNoise1/1(+Noise) -> Mux/2
  AddNoise/1(+Noise) -> Mux/1
  Demux/1 -> AddNoise/1(Signal)
  Demux/3 -> AddNoise2/1(Signal)
  Demux/2 -> AddNoise1/1(Signal)

== system simQuad/Estimator/AddNoise3 ==
  Signal : Inport
  AddNoise : Subsystem
  AddNoise1 : Subsystem
  AddNoise2 : Subsystem
  Demux : Demux  Outputs=3
  Mux : Mux  Inputs=3
  +Noise : Outport
  wires:
  Demux/2 -> AddNoise1/1(Signal)
  Demux/3 -> AddNoise2/1(Signal)
  Demux/1 -> AddNoise/1(Signal)
  AddNoise/1(+Noise) -> Mux/1
  AddNoise1/1(+Noise) -> Mux/2
  AddNoise2/1(+Noise) -> Mux/3
  Signal/1 -> Demux/1
  Mux/1 -> +Noise/1

== system simQuad/Estimator/Mahoney ==
  A : Inport  PortDimensions=[1 3]
  ω : Inport  Port=2  PortDimensions=[1 3]
  Vicon : Inport  Port=3
  q : Inport  Port=4  PortDimensions=[1 4]
  Acceleration Error Estimate : Scope
  Add : Sum  Inputs=+++
  Add1 : Sum
  Constant : Constant  Value=0
  Cross Product : vrlib/Utilities/Cross Product
  Cross Product1 : vrlib/Utilities/Cross Product
  Gain1 : Gain  Gain=0.5
  Integrator : Integrator
  Integrator1 : Integrator  InitialCondition=[1,0,0,0]
  Ki : Gain  Gain=Ki
  Kp : Gain  Gain=Kp
  Mux : Mux  Inputs=2
  Normalize Vector : vrlib/Utilities/Normalize Vector  maxzero=.01
  Normalize Vector1 : vrlib/Utilities/Normalize Vector  maxzero=10e-4
  Total Error Estimate : Scope
  Vicon Error Estimate : Scope
  calc v : MATLAB Function  TreatAsAtomicUnit=on
  calc v3 : MATLAB Function  TreatAsAtomicUnit=on
  quatprod : MATLAB Function  TreatAsAtomicUnit=on
  Quaternion : Outport
  wires:
  A/1 -> Normalize Vector/1
  Constant/1 -> Mux/1
  Add1/1 -> Integrator/1, Kp/1, Total Error Estimate/1
  Ki/1 -> Add/2
  calc v/1(v) -> Cross Product/1, Cross Product1/2
  Add/1 -> Mux/2
  Kp/1 -> Add/1
  Gain1/1 -> Integrator1/1
  quatprod/1(ab) -> Gain1/1
  Mux/1 -> quatprod/2(b)
  Integrator/1 -> Ki/1
  Integrator1/1 -> Normalize Vector1/1
  Normalize Vector1/1 -> Quaternion/1
  q/1 -> calc v/1(q), quatprod/1(a)
  Cross Product/1 -> Acceleration Error Estimate/1, Add1/2
  Vicon/1 -> calc v3/1(q)
  Cross Product1/1 -> Vicon Error Estimate/1, Add1/1
  calc v3/1(v) -> Cross Product1/1
  Normalize Vector/1 -> Cross Product/2
  ω/1 -> Add/3

== system simQuad/Estimator3/AddNoise1 ==
  Signal : Inport
  AddNoise : Subsystem
  AddNoise1 : Subsystem
  AddNoise2 : Subsystem
  Demux : Demux  Outputs=3
  Mux : Mux  Inputs=3
  +Noise : Outport
  wires:
  Demux/2 -> AddNoise1/1(Signal)
  Demux/3 -> AddNoise2/1(Signal)
  Demux/1 -> AddNoise/1(Signal)
  AddNoise/1(+Noise) -> Mux/1
  AddNoise1/1(+Noise) -> Mux/2
  AddNoise2/1(+Noise) -> Mux/3
  Signal/1 -> Demux/1
  Mux/1 -> +Noise/1

== system simQuad/Estimator3/AddNoise3 ==
  Signal : Inport
  AddNoise : Subsystem
  AddNoise1 : Subsystem
  AddNoise2 : Subsystem
  Demux : Demux  Outputs=3
  Mux : Mux  Inputs=3
  +Noise : Outport
  wires:
  Mux/1 -> +Noise/1
  Signal/1 -> Demux/1
  AddNoise2/1(+Noise) -> Mux/3
  AddNoise1/1(+Noise) -> Mux/2
  AddNoise/1(+Noise) -> Mux/1
  Demux/1 -> AddNoise/1(Signal)
  Demux/3 -> AddNoise2/1(Signal)
  Demux/2 -> AddNoise1/1(Signal)

== system simQuad/Estimator3/Mahoney ==
  A : Inport  PortDimensions=[1 3]
  ω : Inport  Port=2  PortDimensions=[1 3]
  Vicon : Inport  Port=3
  q : Inport  Port=4  PortDimensions=[1 4]
  Acceleration Error Estimate : Scope
  Add : Sum  Inputs=+++
  Add1 : Sum
  Constant : Constant  Value=0
  Cross Product : vrlib/Utilities/Cross Product
  Cross Product1 : vrlib/Utilities/Cross Product
  Gain1 : Gain  Gain=0.5
  Integrator : Integrator
  Integrator1 : Integrator  InitialCondition=[1,0,0,0]
  Ki : Gain  Gain=Ki
  Kp : Gain  Gain=Kp
  Mux : Mux  Inputs=2
  Normalize Vector : vrlib/Utilities/Normalize Vector  maxzero=.01
  Normalize Vector1 : vrlib/Utilities/Normalize Vector  maxzero=10e-4
  Total Error Estimate : Scope
  Vicon Error Estimate : Scope
  calc v : MATLAB Function  TreatAsAtomicUnit=on
  calc v3 : MATLAB Function  TreatAsAtomicUnit=on
  quatprod : MATLAB Function  TreatAsAtomicUnit=on
  Quaternion : Outport
  wires:
  ω/1 -> Add/3
  Normalize Vector/1 -> Cross Product/2
  calc v3/1(v) -> Cross Product1/1
  Cross Product1/1 -> Add1/1, Vicon Error Estimate/1
  Vicon/1 -> calc v3/1(q)
  Cross Product/1 -> Add1/2, Acceleration Error Estimate/1
  q/1 -> quatprod/1(a), calc v/1(q)
  Normalize Vector1/1 -> Quaternion/1
  Integrator1/1 -> Normalize Vector1/1
  Integrator/1 -> Ki/1
  Mux/1 -> quatprod/2(b)
  quatprod/1(ab) -> Gain1/1
  Gain1/1 -> Integrator1/1
  Kp/1 -> Add/1
  Add/1 -> Mux/2
  calc v/1(v) -> Cross Product1/2, Cross Product/1
  Ki/1 -> Add/2
  Add1/1 -> Total Error Estimate/1, Kp/1, Integrator/1
  Constant/1 -> Mux/1
  A/1 -> Normalize Vector/1

== system simQuad/Geometric Control/Calc R_des ==
  note: y_B,des
  note: x_C,des
  note: z_B,des
  note: x_B,des
  F_des : Inport
  path_des : Inport  Port=2
  3x3 Cross Product : aerolibutil/3x3 Cross Product
  3x3 Cross Product1 : aerolibutil/3x3 Cross Product
  Gain4 : Gain  Gain=0
  Matrix Concatenate : Concatenate  NumInputs=3  Mode=Multidimensional array  ConcatenateDimension=2
  Mux : Mux  Inputs=3
  Normalization : dspmathops/Normalization  NormType=2-norm  Bias=1e-10  NormOver=Each column  Dimension=1  outputDataTypeStr=Inherit: Same as product output  outputLastDataTypeStr=Inherit: Same as product output  outputMin=[]  outputMax=[]  accumDataTypeStr=Inherit: Same as product output  accumLastDataTypeStr=Inherit: Same as product output  roundingMode=Floor  overflowMode=off
  Normalization1 : dspmathops/Normalization  NormType=2-norm  Bias=1e-10  NormOver=Each column  Dimension=1  outputDataTypeStr=Inherit: Same as product output  outputLastDataTypeStr=Inherit: Same as product output  outputMin=[]  outputMax=[]  accumDataTypeStr=Inherit: Same as product output  accumLastDataTypeStr=Inherit: Same as product output  roundingMode=Floor  overflowMode=off
  Trigonometric Function : Trigonometry
  Trigonometric Function1 : Trigonometry  Operator=cos
  phi_des : Selector  InputPortWidth=4  IndexOptions=Index vector (dialog)  Indices=[4]  OutputSizes=1
  R_des : Outport
  wires:
  3x3 Cross Product1/1 -> Matrix Concatenate/1
  F_des/1 -> Normalization/1
  path_des/1 -> phi_des/1
  Gain4/1 -> Mux/3
  Trigonometric Function1/1 -> Mux/1
  3x3 Cross Product/1 -> Normalization1/1
  Normalization1/1 -> 3x3 Cross Product1/1, Matrix Concatenate/2
  Trigonometric Function/1 -> Mux/2
  Normalization/1 -> 3x3 Cross Product/1, Matrix Concatenate/3, 3x3 Cross Product1/2
  Mux/1 -> 3x3 Cross Product/2
  phi_des/1 -> Gain4/1, Trigonometric Function/1, Trigonometric Function1/1
  Matrix Concatenate/1 -> R_des/1

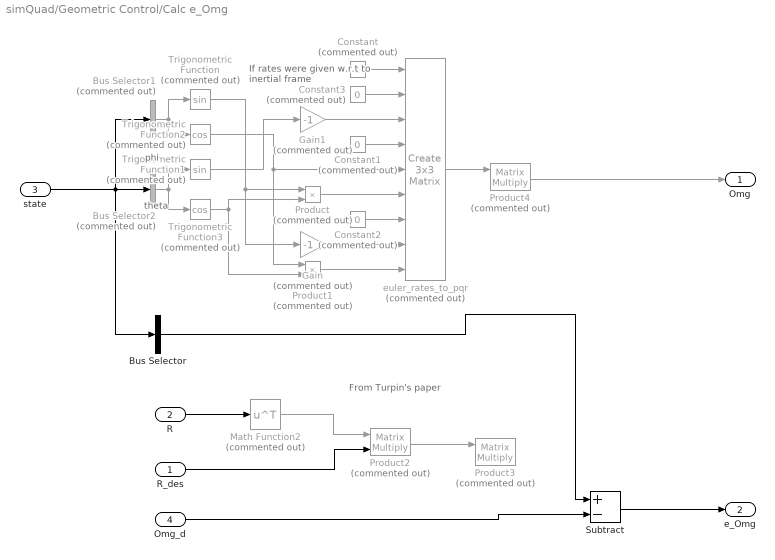
== system simQuad/Geometric Control/Calc e_Omg ==
  note: If rates were given
      | w.r.t to inertial frame
  note: From Turpin's paper
  note: theta
  note: phi
  R_des : Inport
  R : Inport  Port=2
  state : Inport  Port=3
  Omg_d : Inport  Port=4
  Bus Selector : BusSelector  OutputSignals=p,q,r  OutputAsBus=on
  Bus Selector1 : BusSelector  Commented=on  OutputSignals=roll  OutputAsBus=on
  Bus Selector2 : BusSelector  Commented=on  OutputSignals=pitch  OutputAsBus=on
  Constant : Constant  Commented=on
  Constant1 : Constant  Commented=on  Value=0
  Constant2 : Constant  Commented=on  Value=0
  Constant3 : Constant  Commented=on  Value=0
  Gain : Gain  Commented=on  Gain=-1
  Gain1 : Gain  Commented=on  Gain=-1
  Math Function2 : Math  Commented=on  Operator=transpose  SaturateOnIntegerOverflow=on
  Product : Product  Commented=on
  Product1 : Product  Commented=on
  Product2 : Product  Commented=on  Multiplication=Matrix(*)
  Product3 : Product  Commented=on  Multiplication=Matrix(*)
  Product4 : Product  Commented=on  Multiplication=Matrix(*)
  Subtract : Sum  Inputs=+-
  Trigonometric Function : Trigonometry  Commented=on
  Trigonometric Function1 : Trigonometry  Commented=on
  Trigonometric Function2 : Trigonometry  Commented=on  Operator=cos
  Trigonometric Function3 : Trigonometry  Commented=on  Operator=cos
  euler_rates_to_pqr : aerolibutil/Create 3x3 Matrix  Commented=on
  Omg : Outport
  e_Omg : Outport  Port=2
  wires:
  Math Function2/1 -> Product2/1
  R/1 -> Math Function2/1
  Product2/1 -> Product3/1
  R_des/1 -> Product2/2
  Constant/1 -> euler_rates_to_pqr/1
  Constant1/1 -> euler_rates_to_pqr/4
  Constant2/1 -> euler_rates_to_pqr/7
  Bus Selector1/1 -> Trigonometric Function2/1, Trigonometric Function/1
  state/1 -> Bus Selector/1, Bus Selector1/1, Bus Selector2/1
  Bus Selector2/1 -> Trigonometric Function3/1, Trigonometric Function1/1
  Constant3/1 -> euler_rates_to_pqr/2
  Trigonometric Function2/1 -> Product1/1, euler_rates_to_pqr/5
  Trigonometric Function/1 -> Product/1, Gain/1
  Trigonometric Function1/1 -> Gain1/1
  Gain1/1 -> euler_rates_to_pqr/3
  Product/1 -> euler_rates_to_pqr/6
  Trigonometric Function3/1 -> Product/2, Product1/2
  euler_rates_to_pqr/1 -> Product4/1
  Omg_d/1 -> Subtract/2
  Subtract/1 -> e_Omg/1
  Product4/1 -> Omg/1
  Bus Selector/1 -> Subtract/1
  Product1/1 -> euler_rates_to_pqr/9
  Gain/1 -> euler_rates_to_pqr/8

== system simQuad/Geometric Control/Calc e_R ==
  R_des : Inport
  R : Inport  Port=2
  Constant : Constant  Commented=on
  Demux : Demux  Outputs=3
  Divide : Product  Commented=on  Inputs=/*
  Gain1 : Gain  Gain=-1
  Gain4 : Gain  Gain=0.5
  Math Function1 : Math  Operator=transpose  SaturateOnIntegerOverflow=on
  Math Function2 : Math  Operator=transpose  SaturateOnIntegerOverflow=on
  Mux : Mux  Inputs=3
  Product : Product  Multiplication=Matrix(*)
  Product1 : Product  Multiplication=Matrix(*)
  Reshape : Reshape
  Reshape1 : Reshape  Commented=on
  Scope1 : Scope  Commented=on
  Scope2 : Scope  Commented=on
  Sqrt : Sqrt  Commented=on  SaturateOnIntegerOverflow=on
  Sum : Sum  Commented=on  Inputs=++|
  Sum of Elements : Sum  Commented=on  Inputs=+
  Sum3 : Sum  Inputs=+|-
  trace elem : Selector  Commented=on  InputPortWidth=9  IndexOptions=Index vector (dialog)  Indices=[1 5 9]  OutputSizes=1
  vee map : Selector  InputPortWidth=9  IndexOptions=Index vector (dialog)  Indices=[2 3 6]  OutputSizes=1
  e_R : Outport
  wires:
  Math Function2/1 -> Product1/1
  Sum3/1 -> Gain4/1
  Product/1 -> Reshape1/1, Sum3/1
  R/1 -> Product/2, Math Function2/1
  Product1/1 -> Sum3/2
  Math Function1/1 -> Product/1
  vee map/1 -> Demux/1
  Gain4/1 -> Reshape/1
  Reshape/1 -> vee map/1
  R_des/1 -> Product1/2, Math Function1/1
  Demux/1 -> Mux/3
  Demux/3 -> Mux/1
  Gain1/1 -> Mux/2
  Demux/2 -> Gain1/1
  Reshape1/1 -> trace elem/1
  trace elem/1 -> Sum of Elements/1
  Sum of Elements/1 -> Sum/2
  Constant/1 -> Sum/1
  Sum/1 -> Scope1/1, Sqrt/1
  Sqrt/1 -> Divide/1, Scope2/1
  Mux/1 -> e_R/1

== system simQuad/Geometric Control/Motor Mix ==
  T : Inport
  rpy : Inport  Port=2
  Constant : Constant  Value=default_ctl.mix
  Demux : Demux  Outputs=3
  Gain1 : Gain  Gain=ctl.thrust_gain
  Mux : Mux
  Product : Product  Multiplication=Matrix(*)
  Saturation1 : Saturate  UpperLimit=ctl.sat(3,1)  LowerLimit=0
  Saturation2 : Saturate  UpperLimit=ctl.sat(3,1)  LowerLimit=0
  Saturation3 : Saturate  UpperLimit=ctl.sat(1,1)  LowerLimit=ctl.sat(2,1)
  PWM : Outport
  wires:
  Mux/1 -> Product/2
  Product/1 -> Saturation2/1
  Constant/1 -> Product/1
  T/1 -> Gain1/1
  rpy/1 -> Saturation3/1
  Saturation2/1 -> PWM/1
  Saturation1/1 -> Mux/4
  Saturation3/1 -> Demux/1
  Demux/2 -> Mux/2
  Demux/1 -> Mux/1
  Gain1/1 -> Saturation1/1
  Demux/3 -> Mux/3

== system simQuad/Vehicle/PWM 2 Speed ==
  PWM : Inport
  Add{,1..3} (4 alike) : Sum
  Constant{,1..3} (4 alike) : Constant  Value=model.pwm_offset
  Demux : Demux
  Gain{,1..3} (4 alike) : Gain  Gain=model.pwm_gain
  Mux : Mux
  Omega : Outport
  wires:
  Gain/1 -> Add/2
  Constant/1 -> Add/1
  PWM/1 -> Demux/1
  Mux/1 -> Omega/1
  Demux/1 -> Gain/1
  Add/1 -> Mux/1
  Gain1/1 -> Add1/2
  Constant1/1 -> Add1/1
  Gain2/1 -> Add2/2
  Constant2/1 -> Add2/1
  Gain3/1 -> Add3/2
  Constant3/1 -> Add3/1
  Demux/2 -> Gain1/1
  Add1/1 -> Mux/2
  Demux/3 -> Gain2/1
  Add2/1 -> Mux/3
  Demux/4 -> Gain3/1
  Add3/1 -> Mux/4

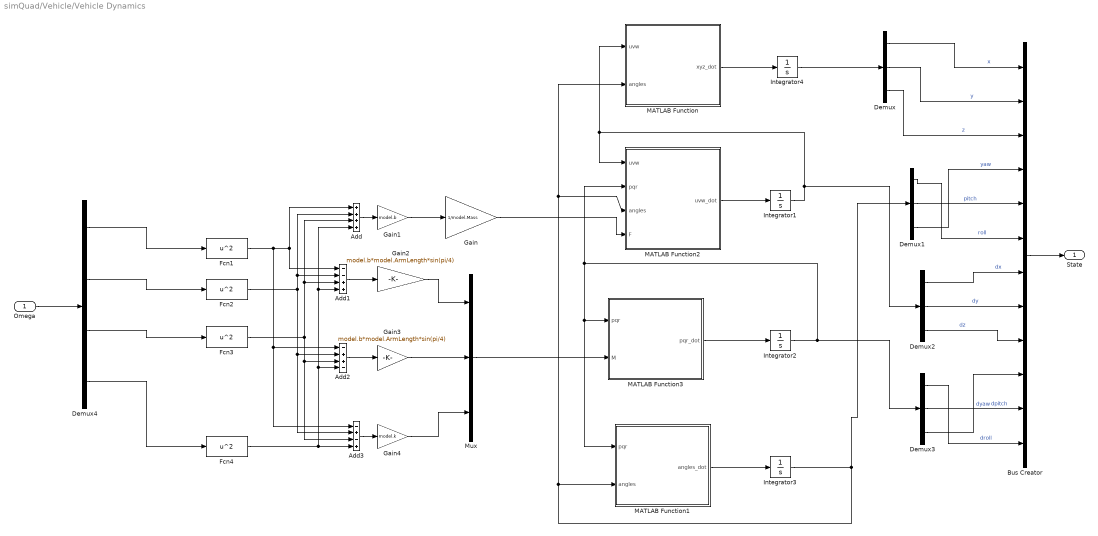
== system simQuad/Vehicle/Vehicle Dynamics ==
  Omega : Inport
  Add : Sum  Inputs=++++
  Add1 : Sum  Inputs=--++
  Add2 : Sum  Inputs=-++-
  Add3 : Sum  Inputs=-+-+
  Bus Creator : BusCreator  Inputs=12
  Demux{,1..3} (4 alike) : Demux  Outputs=3
  Demux4 : Demux
  Fcn{1..4} (4 alike) : Fcn  Expr=u^2
  Gain : Gain  Gain=1/model.Mass
  Gain1 : Gain  Gain=model.b
  Gain2 : Gain  Gain=model.b*model.ArmLength*sin(pi/4)
  Gain3 : Gain  Gain=model.b*model.ArmLength*sin(pi/4)
  Gain4 : Gain  Gain=model.k
  Integrator1 : Integrator  InitialCondition=ic(7:9)
  Integrator2 : Integrator  InitialCondition=ic(10:12)
  Integrator3 : Integrator  InitialCondition=ic(4:6)
  Integrator4 : Integrator  InitialCondition=ic(1:3)
  MATLAB Function : MATLAB Function  TreatAsAtomicUnit=on
  MATLAB Function1 : MATLAB Function  TreatAsAtomicUnit=on
  MATLAB Function2 : MATLAB Function  TreatAsAtomicUnit=on
  MATLAB Function3 : MATLAB Function  TreatAsAtomicUnit=on
  Mux : Mux  Inputs=3
  State : Outport
  wires:
  Gain1/1 -> Gain/1
  Fcn4/1 -> Add/4, Add1/4, Add2/4, Add3/4
  Fcn3/1 -> Add1/3, Add/3, Add2/3, Add3/3
  Fcn2/1 -> Add2/2, Add3/2, Add1/2, Add/2
  Fcn1/1 -> Add/1, Add1/1, Add2/1, Add3/1
  Bus Creator/1 -> State/1
  Add1/1 -> Gain2/1
  Add/1 -> Gain1/1
  Add2/1 -> Gain3/1
  Gain2/1 -> Mux/1
  Gain4/1 -> Mux/3
  Add3/1 -> Gain4/1
  Gain3/1 -> Mux/2
  Gain/1 -> MATLAB Function2/4(F)
  Mux/1 -> MATLAB Function3/2(M)
  MATLAB Function/1(xyz_dot) -> Integrator4/1
  MATLAB Function2/1(uvw_dot) -> Integrator1/1
  MATLAB Function3/1(pqr_dot) -> Integrator2/1
  MATLAB Function1/1(angles_dot) -> Integrator3/1
  Integrator3/1 -> Demux1/1, MATLAB Function/2(angles), MATLAB Function2/3(angles), MATLAB Function1/2(angles)
  Integrator1/1 -> Demux2/1, MATLAB Function/1(uvw), MATLAB Function2/1(uvw)
  Integrator2/1 -> Demux3/1, MATLAB Function2/2(pqr), MATLAB Function1/1(pqr), MATLAB Function3/1(pqr)
  Integrator4/1 -> Demux/1
  Demux/1 -> Bus Creator/1  "x"
  Demux/2 -> Bus Creator/2  "y"
  Demux/3 -> Bus Creator/3  "z"
  Demux1/3 -> Bus Creator/4  "yaw"
  Demux1/1 -> Bus Creator/6  "roll"
  Demux2/1 -> Bus Creator/7  "dx"
  Demux2/3 -> Bus Creator/9  "dz"
  Demux3/3 -> Bus Creator/10  "dyaw"
  Demux3/2 -> Bus Creator/11  "dpitch"
  Demux3/1 -> Bus Creator/12  "droll"
  Demux1/2 -> Bus Creator/5  "pitch"
  Demux2/2 -> Bus Creator/8  "dy"
  Demux4/1 -> Fcn1/1
  Demux4/2 -> Fcn2/1
  Demux4/3 -> Fcn3/1
  Demux4/4 -> Fcn4/1
  Omega/1 -> Demux4/1

== system simQuad/Vehicle3/PWM 2 Speed ==
  PWM : Inport
  Add{,1..3} (4 alike) : Sum
  Constant{,1..3} (4 alike) : Constant  Value=model.pwm_offset
  Demux : Demux
  Gain{,1..3} (4 alike) : Gain  Gain=model.pwm_gain
  Mux : Mux
  Omega : Outport
  wires:
  Add3/1 -> Mux/4
  Demux/4 -> Gain3/1
  Add2/1 -> Mux/3
  Demux/3 -> Gain2/1
  Add1/1 -> Mux/2
  Demux/2 -> Gain1/1
  Constant3/1 -> Add3/1
  Gain3/1 -> Add3/2
  Constant2/1 -> Add2/1
  Gain2/1 -> Add2/2
  Constant1/1 -> Add1/1
  Gain1/1 -> Add1/2
  Add/1 -> Mux/1
  Demux/1 -> Gain/1
  Mux/1 -> Omega/1
  PWM/1 -> Demux/1
  Constant/1 -> Add/1
  Gain/1 -> Add/2
